simulink library "sy202_elevator_library"  (R2016a)
settings: Solver=ode45  StartTime=0.0  StopTime=10.0  RelTol=1e-3
libraries: simulink x1
settings Model: Creator=DeVries  LastModifiedBy=rodrigue
settings DataIOCC: LimitDataPoints=on  SaveFormat=Array
settings HardwareCC: ProdBitPerPointer=32  ProdLargestAtomicFloat=None  ProdIntDivRoundTo=Undefined  ProdEndianess=Unspecified  ProdWordSize=32  ProdHWDeviceType=32-bit Generic
settings ModelReferenceCC: PropagateSignalLabelsOutOfModel=off
settings ConfigComp: CovModelRefEnable=Off

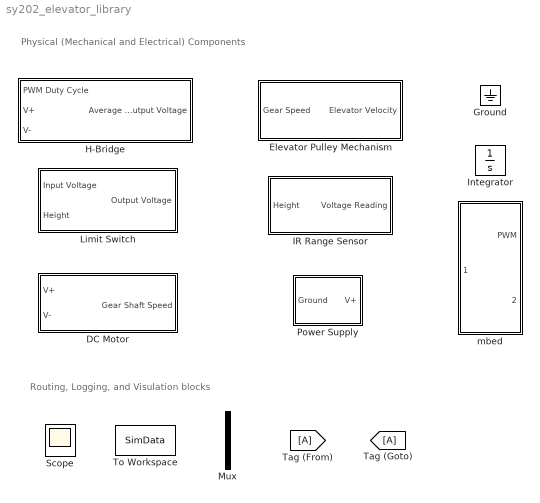
== system sy202_elevator_library ==
  note: Routing, Logging, and Visulation blocks
  note: Physical (Mechanical and Electrical) Components
  DC Motor : Subsystem  mask(DC Motor){ktb=0.0477, Je=1.0081e-05, mass=0.025, Td=0.0029}
      mask prompts: ktb "Transducer Constant"; Je "Moment of Inertia"; mass "Load (Elevator) Mass"; Td "Static Friction"
      mask help:
      | This block represents the dynamics of a direct current motor. The motor has
      | positive and negative voltage input leads and generates the angular
      | velocity of the motor:
      |
      | Inputs:
      |         V+ = Positive reference voltage
      |         V- = Negative reference voltage
      |
      | Output:
      |         Gear Shaft Speed = the rate of rotation of the motor shaft in
      |         rad/s
  Elevator Pulley Mechanism : Subsystem  mask{r_p=0.2015}
      mask prompts: r_p "Pulley Radius"
  Ground : Ground
  H-Bridge : Subsystem  mask(H-Bridge){}
      mask help:
      | The H-bridge block enables control of a DC motor. The H-bridge modifies the voltage level to the DC motor operating voltage switches the current flow to allow directional control.
      |
      | Inputs:
      |     PWM duty cycle: The duty cycle of the PWM motor control signal (from mbed).
      |     V+:             Positive reference voltage
      |     V-:             Negative reference voltage
      |
      | Outputs:
      |     Average Output Voltage: Scaled voltage signal
  IR Range Sensor : Subsystem  mask(Infrared Sensor){noisPow=0.0001, bias=0}
      mask prompts: noisPow "Noise Magnitude"; bias "Bias Error"
      mask help: The block models an infrared range sensor.
  Integrator : Integrator  InitialCondition=10  LimitOutput=on  LowerSaturationLimit=5
  Limit Switch : Subsystem  mask(Elevator Limit Switch(es)){maxHeight=27.125, minHeight=5.75}
      mask prompts: maxHeight "Maximum Height"; minHeight "Minimum Height"
      mask help:
      | This block models the funcitonality of the limit switches on the ES202 elevator setup.  If the height of the elevator car is greater than XX inches or less than YY inches the limit switches are open. Otherwise, the switches are closed.
      |
      | Inputs:
      |         Input Voltage = Voltage into the switch
      |         Height = Height of the elevator car
      |
      | Outputs:
      |         Output Voltage = Voltage on the output side of the switch
      |
      | The parameters set the maximum and minimum heights that open the switches.
  Mux : Mux  Inputs=3
  Power Supply : Subsystem  mask(Power Supply){Vsupply=12}
      mask prompts: Vsupply "Voltage Change"
      mask help:
      | This block models the voltage produced by the power supply. The power supply increases the output voltage above the local ground by an amount specified in the parameter block.
      |
      | Inputs:
      |         Ground = local ground (0 Volts typically)
      |
      | Output:
      |         V+ = output voltage above local ground
      |
      | Parameter:
      |         Voltage Change = Change in voltage generated by the power supply
  Scope : Scope
  To Workspace : ToWorkspace  VariableName=SimData  SaveFormat=Structure With Time  SampleTime=-1
  mbed : Subsystem  mask(Microcontroller Function){DesValue=20, Kp=0.15, Ki=0}
      mask prompts: DesValue "Desired Output Value"; Kp "Proportional Gain (Kp)"; Ki "Integral Gain (Ki)"
      mask help:
      | This block models the implementation of a Proportional-Integral (PI) controller using the mbed microcontroller.  The PI control equation is given by:
      |
      | 	PWM = Kp*error+Ki*(Integral of Error)
      |
      | where the error is  computed as: Desired Output Value - Measured Output.
      |
      | It assumes that the PWM output to DC motor is connected to p21, while the Analog input from sensor is connected to p20. Pin p22 outputs the measured height (i.e., converts sensor's voltage reading to measured output).
      mask Display:
      | image('mbed.jpeg')
      | color('white'); port_label('output',1,'p21')
      | port_label('input',1,'p20')
      | port_label('output',2,'p22')

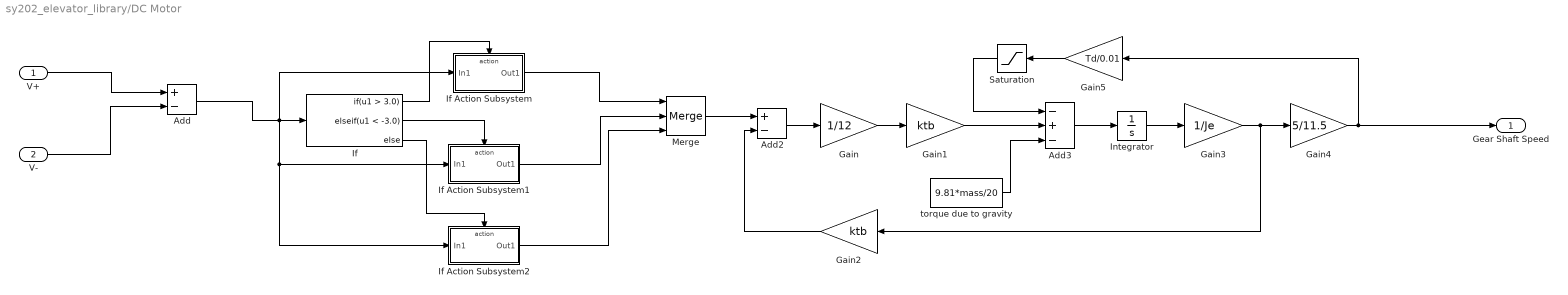
== system sy202_elevator_library/DC Motor ==
  V+ : Inport
  V- : Inport  Port=2
  Add : Sum  Inputs=+-
  Add2 : Sum  Inputs=+-
  Add3 : Sum  Inputs=-+-
  Gain : Gain  Gain=1/12
  Gain1 : Gain  Gain=ktb
  Gain2 : Gain  Gain=ktb
  Gain3 : Gain  Gain=1/Je
  Gain4 : Gain  Gain=5/11.5
  Gain5 : Gain  Gain=Td/0.01
  If : If  IfExpression=u1 > 3.0  ElseIfExpressions=u1 < -3.0
  If Action Subsystem : Subsystem  TreatAsAtomicUnit=on
  If Action Subsystem1 : Subsystem  TreatAsAtomicUnit=on
  If Action Subsystem2 : Subsystem  TreatAsAtomicUnit=on
  Integrator : Integrator
  Merge : Merge  Inputs=3
  Saturation : Saturate  UpperLimit=Td  LowerLimit=-Td
  torque due to gravity : Constant  Value=9.81*mass/20
  Gear Shaft Speed : Outport
  wires:
  Add/1 -> If Action Subsystem/1(In1), If Action Subsystem1/1(In1), If Action Subsystem2/1(In1), If/1
  Merge/1 -> Add2/1
  If/3 -> If Action Subsystem2/Action
  If/1 -> If Action Subsystem/Action
  If Action Subsystem2/1(Out1) -> Merge/3
  If Action Subsystem1/1(Out1) -> Merge/2
  If Action Subsystem/1(Out1) -> Merge/1
  If/2 -> If Action Subsystem1/Action
  V+/1 -> Add/1
  V-/1 -> Add/2
  Add2/1 -> Gain/1
  Gain/1 -> Gain1/1
  Integrator/1 -> Gain3/1
  Gain3/1 -> Gain4/1, Gain2/1
  Gain1/1 -> Add3/2
  Saturation/1 -> Add3/1
  Gain5/1 -> Saturation/1
  Gain2/1 -> Add2/2
  Add3/1 -> Integrator/1
  Gain4/1 -> Gain5/1, Gear Shaft Speed/1
  torque due to gravity/1 -> Add3/3

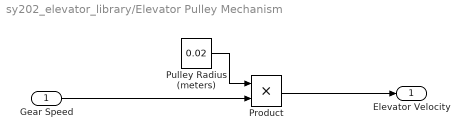
== system sy202_elevator_library/Elevator Pulley Mechanism ==
  Gear Speed : Inport
  Product : Product
  Pulley Radius (meters) : Constant  Value=0.02
  Elevator Velocity : Outport
  wires:
  Gear Speed/1 -> Product/2
  Pulley Radius (meters)/1 -> Product/1
  Product/1 -> Elevator Velocity/1

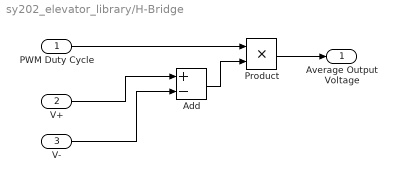
== system sy202_elevator_library/H-Bridge ==
  PWM Duty Cycle : Inport
  V+ : Inport  Port=2
  V- : Inport  Port=3
  Add : Sum  Inputs=+-
  Product : Product
  Average Output Voltage : Outport
  wires:
  Product/1 -> Average Output Voltage/1
  PWM Duty Cycle/1 -> Product/1
  Add/1 -> Product/2
  V+/1 -> Add/1
  V-/1 -> Add/2

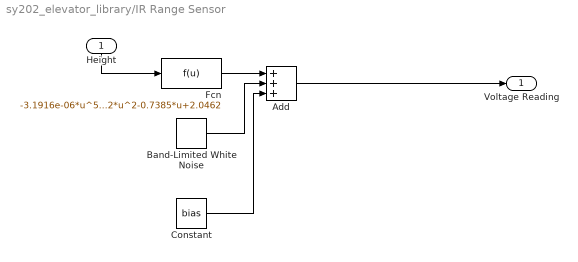
== system sy202_elevator_library/IR Range Sensor ==
  Height : Inport
  Add : Sum  Inputs=+++
  Band-Limited White Noise : simulink/Sources/Band-Limited White Noise  Cov=[noisPow]  Ts=0.1  seed=[23341]
  Constant : Constant  Value=bias
  Fcn : Fcn  Expr=-3.1916e-06*u^5+2.5367e-04*u^4-7.6155e-03*u^3+0.1092*u^2-0.7385*u+2.0462
  Voltage Reading : Outport
  wires:
  Add/1 -> Voltage Reading/1
  Band-Limited White Noise/1 -> Add/2
  Fcn/1 -> Add/1
  Height/1 -> Fcn/1
  Constant/1 -> Add/3

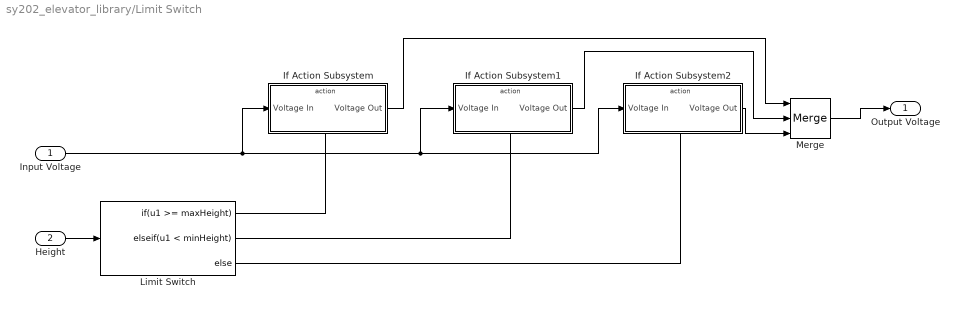
== system sy202_elevator_library/Limit Switch ==
  Input Voltage : Inport
  Height : Inport  Port=2
  If Action Subsystem : Subsystem  TreatAsAtomicUnit=on
  If Action Subsystem1 : Subsystem  TreatAsAtomicUnit=on
  If Action Subsystem2 : Subsystem  TreatAsAtomicUnit=on
  Limit Switch : If  IfExpression=u1 >= maxHeight  ElseIfExpressions=u1 < minHeight
  Merge : Merge  Inputs=3
  Output Voltage : Outport
  wires:
  Height/1 -> Limit Switch/1
  Input Voltage/1 -> If Action Subsystem2/1(Voltage In), If Action Subsystem1/1(Voltage In), If Action Subsystem/1(Voltage In)
  Limit Switch/3 -> If Action Subsystem2/Action
  Limit Switch/2 -> If Action Subsystem1/Action
  Limit Switch/1 -> If Action Subsystem/Action
  If Action Subsystem/1(Voltage Out) -> Merge/1
  If Action Subsystem1/1(Voltage Out) -> Merge/2
  If Action Subsystem2/1(Voltage Out) -> Merge/3
  Merge/1 -> Output Voltage/1

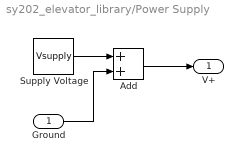
== system sy202_elevator_library/Power Supply ==
  Ground : Inport
  Add : Sum
  Supply Voltage : Constant  Value=Vsupply
  V+ : Outport
  wires:
  Supply Voltage/1 -> Add/1
  Add/1 -> V+/1
  Ground/1 -> Add/2

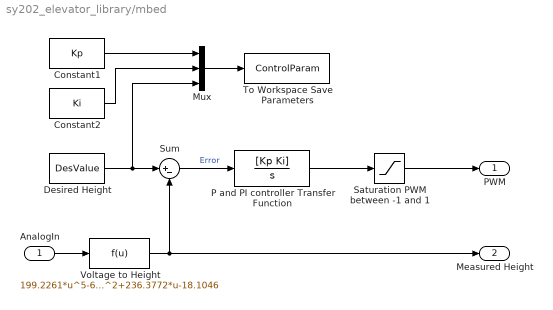
== system sy202_elevator_library/mbed ==
  AnalogIn : Inport
  Constant1 : Constant  Value=Kp
  Constant2 : Constant  Value=Ki
  Desired Height : Constant  Value=DesValue
  Mux : Mux  Inputs=3
  P and PI controller Transfer Function : TransferFcn  Numerator=[Kp Ki]  Denominator=[1 0]
  Saturation PWM between -1 and 1 : Saturate  UpperLimit=1  LowerLimit=-1
  Sum : Sum  Inputs=|+-
  To Workspace Save Parameters : ToWorkspace  VariableName=ControlParam  SaveFormat=Structure  SampleTime=-1
      settings: MaxDataPoints=1
  Voltage to Height : Fcn  Expr=199.2261*u^5-635.0808*u^4+854.2399*u^3-607.8445*u^2+236.3772*u-18.1046
  PWM : Outport
  Measured Height : Outport  Port=2
  wires:
  Saturation PWM between -1 and 1/1 -> PWM/1
  P and PI controller Transfer Function/1 -> Saturation PWM between -1 and 1/1
  Desired Height/1 -> Mux/3, Sum/1
  Sum/1 -> P and PI controller Transfer Function/1  "Error"
  Voltage to Height/1 -> Sum/2, Measured Height/1
  AnalogIn/1 -> Voltage to Height/1
  Mux/1 -> To Workspace Save Parameters/1
  Constant1/1 -> Mux/1
  Constant2/1 -> Mux/2

== system sy202_elevator_library/DC Motor/If Action Subsystem ==
  In1 : Inport
  Action Port : ActionPort
  Out1 : Outport
  wires:
  In1/1 -> Out1/1

== system sy202_elevator_library/DC Motor/If Action Subsystem1 ==
  In1 : Inport
  Action Port : ActionPort
  Out1 : Outport
  wires:
  In1/1 -> Out1/1

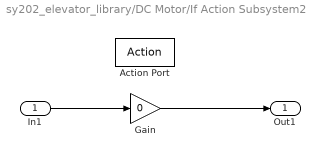
== system sy202_elevator_library/DC Motor/If Action Subsystem2 ==
  In1 : Inport
  Action Port : ActionPort
  Gain : Gain  Gain=0
  Out1 : Outport
  wires:
  In1/1 -> Gain/1
  Gain/1 -> Out1/1

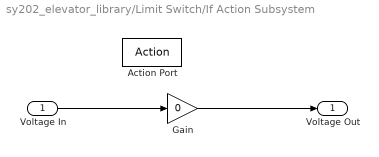
== system sy202_elevator_library/Limit Switch/If Action Subsystem ==
  Voltage In : Inport
  Action Port : ActionPort
  Gain : Gain  Gain=0
  Voltage Out : Outport
  wires:
  Voltage In/1 -> Gain/1
  Gain/1 -> Voltage Out/1

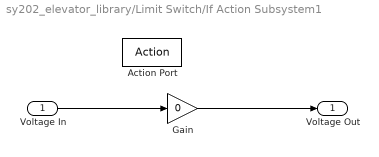
== system sy202_elevator_library/Limit Switch/If Action Subsystem1 ==
  Voltage In : Inport
  Action Port : ActionPort
  Gain : Gain  Gain=0
  Voltage Out : Outport
  wires:
  Voltage In/1 -> Gain/1
  Gain/1 -> Voltage Out/1

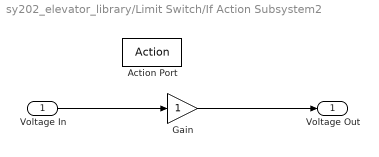
== system sy202_elevator_library/Limit Switch/If Action Subsystem2 ==
  Voltage In : Inport
  Action Port : ActionPort
  Gain : Gain
  Voltage Out : Outport
  wires:
  Voltage In/1 -> Gain/1
  Gain/1 -> Voltage Out/1
